simulink model "sampleModel1494"  (R2023a)
settings: Solver=VariableStepAuto  StartTime=0.0  StopTime=10.0  RelTol=1e-3
libraries: simulink x2, hdlsllib x1
settings Model: Creator=user1  LastModifiedBy=user1

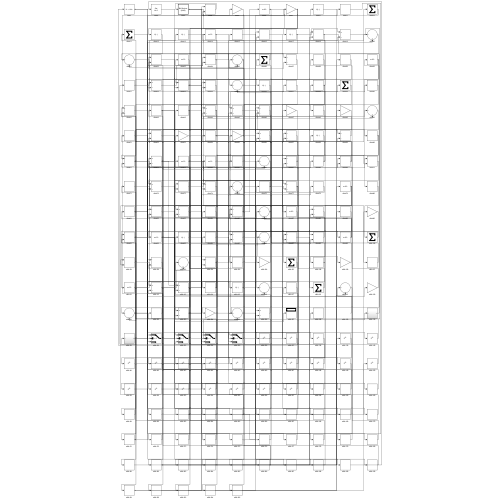
[thumbnail: Simulink's stored preview of the top-level diagram]
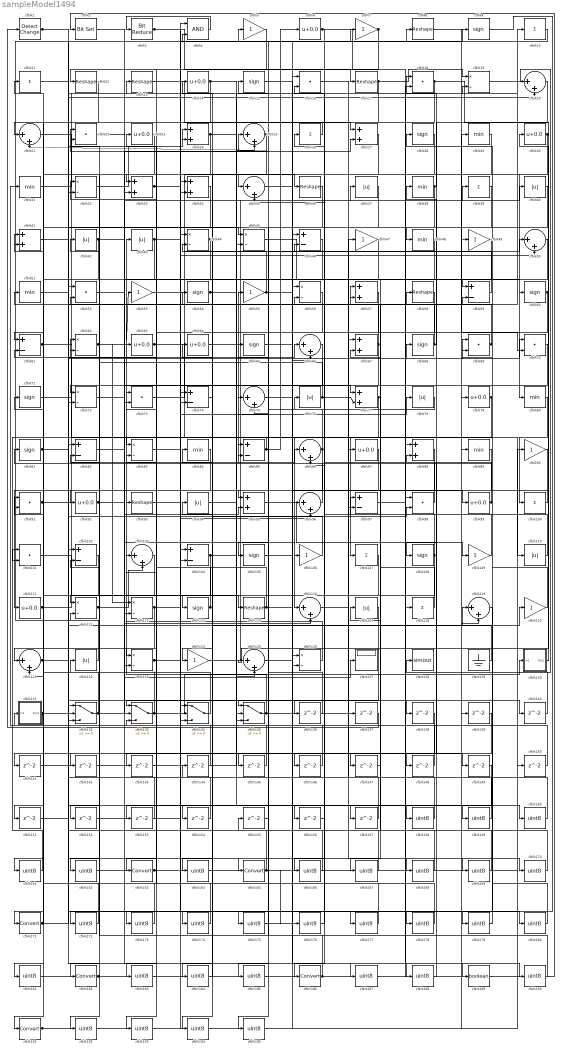
== system sampleModel1494 ==
  cfblk1 : simulink/Logic and Bit Operations/Detect Change  vinit=0  OutDataTypeStr=boolean
      settings: LibrarySourceBlock=|
      | hdlsllib/Logic and Bit
      | Operations/Detect
      | Change
  cfblk{10..11,26,39,100,107,118} (7 alike) : Sum  Inputs=+
  cfblk{16,18,22,52,69..70,73,91,98,101} (10 alike) : DotProduct  OutDataTypeStr=Inherit: Inherit via internal rule
  cfblk{46,59,61,74,82,85,97,102,104} (9 alike) : Sum  Inputs=+-
  cfblk{20..21,25,35,50,66,75,86,96,103,116,119,121,125} (14 alike) : Sum  Inputs=|++
  cfblk{9,15,28,54,60,65,68,71,81,105,108,114} (12 alike) : Signum
  cfblk{5,7,47,49,53,55,90,106,109,120,124} (11 alike) : Gain
  cfblk{37,40,42..43,76,78,94,110,117,122} (10 alike) : Abs  SaturateOnIntegerOverflow=off
  cfblk{6,14,23,30,63..64,79,87,92,99,111} (11 alike) : Bias  Bias=0.0  SaturateOnIntegerOverflow=off
  cfblk{19,32,44..45,56,62,72,83,112..113,123,126} (12 alike) : Product  Inputs=*/  RndMeth=Zero  SaturateOnIntegerOverflow=on
  cfblk{8,12..13,17,36,58,93,115} (8 alike) : Reshape
  cfblk127 : Display
  cfblk128 : ToWorkspace  VariableName=simout  SaveFormat=Timeseries  SampleTime=-1
  cfblk129 : Ground
  cfblk130 : Subsystem
      settings: LibrarySourceBlock=|
      | hdlsllib/Ports &
      | Subsystems/Subsystem
  cfblk131 : Subsystem
      settings: LibrarySourceBlock=|
      | hdlsllib/Ports &
      | Subsystems/Subsystem
  cfblk{132..135} (4 alike) : Switch  SaturateOnIntegerOverflow=off  InputSameDT=off
  cfblk{136..157} (22 alike) : Delay  SampleTime=1
  cfblk{158..162,164,166..170,172..181,183..185,187..188,190,192..195} (31 alike) : DataTypeConversion  OutDataTypeStr=uint8  SaturateOnIntegerOverflow=off  RndMeth=Floor
  cfblk{163,165,171,182,186,191} (6 alike) : DataTypeConversion  SaturateOnIntegerOverflow=off  RndMeth=Floor
  cfblk189 : DataTypeConversion  OutDataTypeStr=boolean  SaturateOnIntegerOverflow=off  RndMeth=Floor
  cfblk2 : simulink/Logic and Bit Operations/Bit Set  iBit=0
      settings: LibrarySourceBlock=|
      | hdlsllib/Logic and Bit
      | Operations/Bit Set
  cfblk{24,27,33..34,41,57,67,77,88,95} (10 alike) : Sum
  cfblk{29,31,38,48,51,80,84,89} (8 alike) : MinMax
  cfblk3 : hdlsllib/Logic and Bit Operations/Bit Reduce  mode=AND
  cfblk4 : Logic  AllPortsSameDT=off  OutDataTypeStr=boolean
  wires:
  cfblk124/1 -> cfblk39/1
  cfblk32/1 -> cfblk24/1
  cfblk101/1 -> cfblk115/1
  cfblk53/1 -> cfblk36/1
  cfblk135/1 -> cfblk43/1, cfblk47/1
  cfblk84/1 -> cfblk163/1
  cfblk122/1 -> cfblk8/1
  cfblk115/1 -> cfblk61/2, cfblk138/1
  cfblk30/1 -> cfblk80/1, cfblk35/1
  cfblk120/1 -> cfblk28/1
  cfblk111/1 -> cfblk69/1, cfblk20/2
  cfblk18/1 -> cfblk125/1, cfblk32/2
  cfblk62/1 -> cfblk53/1, cfblk113/1, cfblk27/2
  cfblk88/1 -> cfblk186/1
  cfblk34/1 -> cfblk191/1
  cfblk78/1 -> cfblk76/1
  cfblk1/1 -> cfblk133/2, cfblk159/1
  cfblk132/1 -> cfblk71/1, cfblk40/1, cfblk127/1
  cfblk20/1 -> cfblk108/1
  cfblk126/1 -> cfblk93/1
  cfblk26/1 -> cfblk21/1
  cfblk54/1 -> cfblk19/2, cfblk146/1
  cfblk87/1 -> cfblk111/1
  cfblk85/1 -> cfblk83/1, cfblk6/1
  cfblk63/1 -> cfblk107/1, cfblk87/1
  cfblk91/1 -> cfblk55/1, cfblk5/1
  cfblk25/1 -> cfblk21/2, cfblk33/1
  cfblk21/1 -> cfblk118/1
  cfblk110/1 -> cfblk85/1
  cfblk4/1 -> cfblk3/1
  cfblk23/1 -> cfblk132/2
  cfblk14/1 -> cfblk25/2, cfblk33/2
  cfblk15/1 -> cfblk56/1
  cfblk100/1 -> cfblk92/1
  cfblk114/1 -> cfblk62/1, cfblk32/1
  cfblk60/1 -> cfblk124/1, cfblk157/1
  cfblk92/1 -> cfblk116/2, cfblk106/1, cfblk136/1
  cfblk40/1 -> cfblk48/1
  cfblk17/1 -> cfblk19/1, cfblk134/3
  cfblk104/1 -> cfblk37/1, cfblk193/1
  cfblk73/1 -> cfblk50/1
  cfblk95/1 -> cfblk109/1
  cfblk118/1 -> cfblk97/1
  cfblk3/1 -> cfblk17/1, cfblk50/2, cfblk135/2
  cfblk39/1 -> cfblk97/2
  cfblk102/1 -> cfblk171/1
  cfblk68/1 -> cfblk38/1, cfblk41/1
  cfblk80/1 -> cfblk100/1
  cfblk45/1 -> cfblk59/1
  cfblk5/1 -> cfblk12/1
  cfblk67/1 -> cfblk11/1, cfblk123/2
  cfblk12/1 -> cfblk121/1
  cfblk24/1 -> cfblk27/1, cfblk142/1
  cfblk134/1 -> cfblk91/1
  cfblk6/1 -> cfblk98/1, cfblk96/1
  cfblk19/1 -> cfblk128/1
  cfblk117/1 -> cfblk133/1
  cfblk74/1 -> cfblk114/1
  cfblk43/1 -> cfblk151/1, cfblk175/1
  cfblk47/1 -> cfblk105/1
  cfblk64/1 -> cfblk20/1
  cfblk69/1 -> cfblk58/1, cfblk41/2
  cfblk75/1 -> cfblk9/1
  cfblk81/1 -> cfblk70/1, cfblk57/2
  cfblk41/1 -> cfblk24/2
  cfblk96/1 -> cfblk73/1
  cfblk77/1 -> cfblk95/1, cfblk167/1
  cfblk107/1 -> cfblk112/1
  cfblk133/1 -> cfblk130/1(In1), cfblk112/2
  cfblk33/1 -> cfblk7/1, cfblk135/3
  cfblk79/1 -> cfblk116/1, cfblk101/2, cfblk148/1
  cfblk31/1 -> cfblk10/1
  cfblk38/1 -> cfblk18/1, cfblk86/2, cfblk143/1
  cfblk86/1 -> cfblk22/1, cfblk185/1
  cfblk52/1 -> cfblk165/1
  cfblk56/1 -> cfblk75/2
  cfblk59/1 -> cfblk15/1
  cfblk83/1 -> cfblk68/1
  cfblk13/1 -> cfblk125/2
  cfblk42/1 -> cfblk77/1, cfblk61/1, cfblk60/1
  cfblk36/1 -> cfblk135/1
  cfblk8/1 -> cfblk70/2
  cfblk71/1 -> cfblk126/1
  cfblk113/1 -> cfblk78/1, cfblk121/2, cfblk96/2
  cfblk76/1 -> cfblk77/2, cfblk22/2
  cfblk11/1 -> cfblk45/1
  cfblk10/1 -> cfblk4/2
  cfblk131/1(Out1) -> cfblk31/1, cfblk66/1, cfblk120/1
  cfblk61/1 -> cfblk110/1, cfblk188/1
  cfblk129/1 -> cfblk94/1
  cfblk123/1 -> cfblk104/2, cfblk86/1
  cfblk112/1 -> cfblk103/2, cfblk95/2, cfblk152/1
  cfblk108/1 -> cfblk35/2, cfblk154/1
  cfblk55/1 -> cfblk44/2, cfblk99/1
  cfblk130/1(Out1) -> cfblk30/1
  cfblk66/1 -> cfblk74/2
  cfblk7/1 -> cfblk123/1, cfblk113/2, cfblk183/1
  cfblk121/1 -> cfblk13/1, cfblk98/2
  cfblk106/1 -> cfblk14/1
  cfblk44/1 -> cfblk72/1, cfblk73/2
  cfblk99/1 -> cfblk57/1, cfblk85/2, cfblk81/1
  cfblk109/1 -> cfblk26/1
  cfblk98/1 -> cfblk54/1
  cfblk49/1 -> cfblk182/1
  cfblk103/1 -> cfblk132/3
  cfblk136/1 -> cfblk4/1
  cfblk116/1 -> cfblk137/1
  cfblk137/1 -> cfblk1/1
  cfblk65/1 -> cfblk140/1
  cfblk140/1 -> cfblk59/2
  cfblk27/1 -> cfblk141/1
  cfblk141/1 -> cfblk44/1
  cfblk142/1 -> cfblk45/2
  cfblk143/1 -> cfblk134/2
  cfblk144/1 -> cfblk134/1
  cfblk22/1 -> cfblk145/1
  cfblk145/1 -> cfblk83/2
  cfblk146/1 -> cfblk25/1
  cfblk50/1 -> cfblk147/1
  cfblk147/1 -> cfblk67/2
  cfblk148/1 -> cfblk133/3
  cfblk93/1 -> cfblk149/1
  cfblk150/1 -> cfblk91/2
  cfblk152/1 -> cfblk74/1
  cfblk58/1 -> cfblk153/1
  cfblk153/1 -> cfblk132/1
  cfblk154/1 -> cfblk62/2
  cfblk155/1 -> cfblk75/1
  cfblk90/1 -> cfblk156/1
  cfblk156/1 -> cfblk56/2
  cfblk157/1 -> cfblk42/1
  cfblk82/1 -> cfblk158/1
  cfblk158/1 -> cfblk67/1
  cfblk159/1 -> cfblk82/1
  cfblk94/1 -> cfblk160/1
  cfblk160/1 -> cfblk82/2
  cfblk139/1 -> cfblk161/1
  cfblk161/1 -> cfblk101/1
  cfblk70/1 -> cfblk162/1
  cfblk162/1 -> cfblk139/1
  cfblk163/1 -> cfblk90/1, cfblk23/1
  cfblk57/1 -> cfblk164/1
  cfblk164/1 -> cfblk84/1
  cfblk165/1 -> cfblk155/1, cfblk64/1, cfblk176/1
  cfblk28/1 -> cfblk166/1
  cfblk166/1 -> cfblk52/1
  cfblk167/1 -> cfblk52/2
  cfblk16/1 -> cfblk168/1
  cfblk168/1 -> cfblk117/1
  cfblk151/1 -> cfblk169/1
  cfblk169/1 -> cfblk16/1
  cfblk72/1 -> cfblk170/1
  cfblk170/1 -> cfblk16/2
  cfblk171/1 -> cfblk72/2, cfblk131/1(In1)
  cfblk9/1 -> cfblk172/1
  cfblk172/1 -> cfblk102/1
  cfblk149/1 -> cfblk173/1
  cfblk173/1 -> cfblk102/2
  cfblk46/1 -> cfblk174/1
  cfblk174/1 -> cfblk63/1
  cfblk175/1 -> cfblk46/1
  cfblk176/1 -> cfblk46/2
  cfblk51/1 -> cfblk177/1
  cfblk177/1 -> cfblk103/1
  cfblk105/1 -> cfblk178/1
  cfblk178/1 -> cfblk51/1
  cfblk119/1 -> cfblk179/1
  cfblk179/1 -> cfblk69/2
  cfblk35/1 -> cfblk180/1
  cfblk180/1 -> cfblk119/1
  cfblk48/1 -> cfblk181/1
  cfblk181/1 -> cfblk119/2
  cfblk182/1 -> cfblk66/2, cfblk18/2
  cfblk183/1 -> cfblk49/1
  cfblk89/1 -> cfblk184/1
  cfblk184/1 -> cfblk144/1
  cfblk185/1 -> cfblk89/1
  cfblk186/1 -> cfblk65/1, cfblk122/1
  cfblk125/1 -> cfblk187/1
  cfblk187/1 -> cfblk88/1
  cfblk188/1 -> cfblk88/2
  cfblk97/1 -> cfblk189/1
  cfblk189/1 -> cfblk2/1
  cfblk2/1 -> cfblk190/1
  cfblk190/1 -> cfblk104/1
  cfblk191/1 -> cfblk126/2, cfblk79/1
  cfblk138/1 -> cfblk192/1
  cfblk192/1 -> cfblk34/1
  cfblk193/1 -> cfblk34/2
  cfblk29/1 -> cfblk194/1
  cfblk194/1 -> cfblk150/1
  cfblk37/1 -> cfblk195/1
  cfblk195/1 -> cfblk29/1

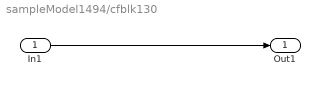
== system sampleModel1494/cfblk130 ==
  In1 : Inport
  Out1 : Outport
  wires:
  In1/1 -> Out1/1

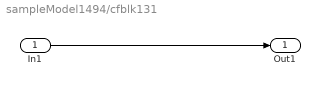
== system sampleModel1494/cfblk131 ==
  In1 : Inport
  Out1 : Outport
  wires:
  In1/1 -> Out1/1
